simulink model "testing"  (R2021a)
settings: Solver=VariableStepAuto  StartTime=0.0  StopTime=10.0  RelTol=1e-3
undefined symbols (not defined in the file or in its folder): weird_test
settings Model: Creator=nathanielgoldfarb  LastModifiedBy=nathanielgoldfarb

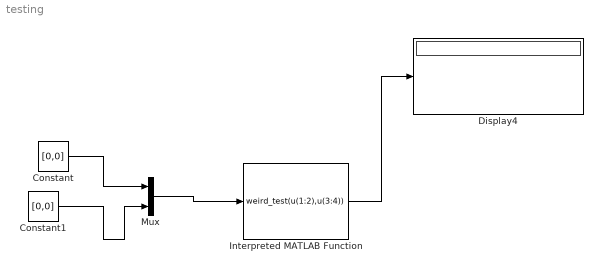
== system testing ==
  Constant : Constant  Value=[0,0]
  Constant1 : Constant  Value=[0,0]
  Display4 : Display
  Interpreted MATLAB Function : MATLABFcn  MATLABFcn=weird_test(u(1:2),u(3:4))  Output1D=off
  Mux : Mux  Inputs=2
  wires:
  Mux/1 -> Interpreted MATLAB Function/1
  Constant/1 -> Mux/1
  Constant1/1 -> Mux/2
  Interpreted MATLAB Function/1 -> Display4/1
